simulink model "color_palette_v1"  (Simulink 7.6)
settings: Solver=FixedStepDiscrete  StartTime=0.0  StopTime=0  FixedStep=1/30  RelTol=1e-3
undefined symbols (not defined in the file or in its folder): a_halfrange, a_offset, b_halfrange, b_offset, jet, Rec, ref_colors, refColorSelect, SDTV
libraries: vipconversions x1, vipsnks x1
settings Model: Creator=auvt  LastModifiedBy=auvt
settings RTWCC: TargetLang=C++

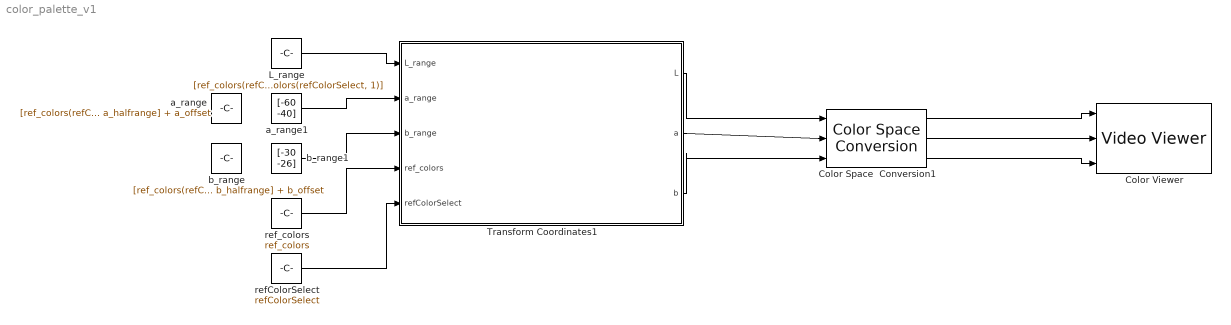
== system color_palette_v1 ==
  Color Space  Conversion1 : vipconversions/Color Space  Conversion  conversion=Obsolete  conversionActive=L*a*b* to sR'G'B'  wp_str=D50  rec=Rec. 601 (SDTV)  sys=1125/60/2:1  imagePorts=Separate color signals
  Color Viewer : vipsnks/Video Viewer  DialogControllerArgs=DataTag1  inputType=Obsolete7b  imagePorts=Separate color signals  useColorMap=off  colormapValue=jet(256)  specRange=off  minInputVal=0  maxInputVal=255  FigPos=[2117 436 410 300]  AxisZoom=on  trueSizedOnce=off  OpenAtMdlStart=on
  L_range : Constant  Value=[ref_colors(refColorSelect, 1) ref_colors(refColorSelect, 1)]  SampleTime=-1
  Transform Coordinates1 : Stateflow chart  TreatAsAtomicUnit=on  SystemSampleTime=[1/30 0]
  a_range : Constant  Value=[ref_colors(refColorSelect, 2) ref_colors(refColorSelect, 2)] + [-a_halfrange, a_halfrange] + a_offset  SampleTime=-1
  a_range1 : Constant  Value=[-60 -40]  SampleTime=-1
  b_range : Constant  Value=[ref_colors(refColorSelect, 3) ref_colors(refColorSelect, 3)] + [-b_halfrange, b_halfrange] + b_offset  SampleTime=-1
  b_range1 : Constant  Value=[-30 -26]  SampleTime=-1
  refColorSelect : Constant  Value=refColorSelect  SampleTime=-1
  ref_colors : Constant  Value=ref_colors  SampleTime=-1
  wires:
  Transform Coordinates1/1(L) -> Color Space  Conversion1/1
  Transform Coordinates1/2(a) -> Color Space  Conversion1/2
  Transform Coordinates1/3(b) -> Color Space  Conversion1/3
  Color Space  Conversion1/1 -> Color Viewer/1
  Color Space  Conversion1/2 -> Color Viewer/2
  Color Space  Conversion1/3 -> Color Viewer/3
  L_range/1 -> Transform Coordinates1/1(L_range)
  ref_colors/1 -> Transform Coordinates1/4(ref_colors)
  refColorSelect/1 -> Transform Coordinates1/5(refColorSelect)
  a_range1/1 -> Transform Coordinates1/2(a_range)
  b_range1/1 -> Transform Coordinates1/3(b_range)

== matlab function Transform Coordinates1 ==
  data: L_range input double; a_range input double; b_range input double; L output double; a output double; b output double; ref_colors input double; refColorSelect input double
function [L, a, b] = makePalette(L_range, a_range, b_range, ref_colors, refColorSelect)


% Initialize
rows = 200;
cols = 200;

L = zeros(rows, cols);
a = zeros(rows, cols);
b = zeros(rows, cols);


% Display the valid color range gradient
for r = 1:rows
    for c = 1:cols
        
        L(r,c) = L_range(1);
        a(r,c) = a_range(1) + (a_range(2) - a_range(1) )*( (r-1)/(rows-1) );
        b(r,c) = b_range(1) + (b_range(2) - b_range(1) )*( (c-1)/(cols-1) );
        
    end
end


% Place a box in the center of the viewing area with the refColorSelect'th
%   color in ref_colors
for r = 90:110
    for c = 90:110
        L(r,c) = ref_colors(refColorSelect, 1);
        a(r,c) = ref_colors(refColorSelect, 2);
        b(r,c) = ref_colors(refColorSelect, 3);
    end
end


return
